simulink model "cv_model_50F"  (R2023a)
settings: Solver=ode23t  StartTime=0  StopTime=5040  FixedStep=0.0005  MaxStep=.01  RelTol=1e-4
model workspace (MAT data in the model file):
  test = 0
values from neighbouring files (symbols this model uses):
  A_cheb_09_1 = [-9.45889157397 1 0 0 0 0 0 0 0 -116.684730988 0 1 ... (81 elements, 9x9)]    [input_reflex_filters.mat]
  B_cheb_09_1 = [1 0 0 0 0 0 0 0 0]    [input_reflex_filters.mat]
  C_cheb_09_1 = [0 0 0 0 0 0 0 0 151338.279895]    [input_reflex_filters.mat]
libraries: SignalEditorBlockLib x4, simulink_extras x2
(part 1 of 3)
settings Model: ExtModeTrigMode=oneshot  Creator=samar  LastModifiedBy=Rich
settings SolverCC: AlgebraicLoopSolver=TrustRegion
settings DataIOCC: SaveFormat=Array  SignalLoggingSaveFormat=ModelDataLogs  ReturnWorkspaceOutputs=off  SignalLoggingName=sigsOut
settings OptimizationCC: BooleanDataType=off  InitFltsAndDblsToZero=on  LifeSpan=inf
settings DebuggingCC: ConsistencyChecking=warning  SaveWithParameterizedLinksMsg=none  UnderspecifiedInitializationDetection=Classic  MergeDetectMultiDrivingBlocksExec=none  SignalResolutionControl=TryResolveAllWithWarning  MultiTaskDSMMsg=warning  MultiTaskCondExecSysMsg=none  FcnCallInpInsideContextMsg=warning  SFUnexpectedBacktrackingDiag=warning  SFNoUnconditionalDefaultTransitionDiag=warning  SFExecutionAtInitializationDiag=none  ArithmeticOperatorsInVariantConditions=warning
settings HardwareCC: ProdBitPerPointer=32  ProdBitPerSizeT=32  ProdBitPerPtrDiffT=32  ProdLargestAtomicFloat=None  ProdIntDivRoundTo=Undefined  ProdEndianess=Unspecified  ProdWordSize=32  ProdHWDeviceType=32-bit Generic  TargetUnknown=on
settings ModelReferenceCC: EnableRefExpFcnMdlSchedulingChecks=on  PropagateSignalLabelsOutOfModel=off
settings SFSimCC: SimUseLocalCustomCode=off  CustomCodeUndefinedFunction=UseInterfaceOnly
settings RTWCC: TemplateMakefile=grt_unix.tmf  RTWUseLocalCustomCode=off  DLArmComputeVersion=19.05
settings CodeAppCC: StateflowObjectComments=on
settings GRTTargetCC: TargetFcnLib=ansi_tfl_tmw.mat  TargetLangStandard=C89/C90 (ANSI)  ModelReferenceCompliant=off  CombineOutputUpdateFcns=off  MatFileLogging=off  GRTInterface=on
settings ConfigComp: CovMetricSettings=dw  CovSaveCumulativeToWorkspaceVar=on  CovSaveSingleToWorkspaceVar=on  CovExternalEMLEnable=off  CovSFcnEnable=off

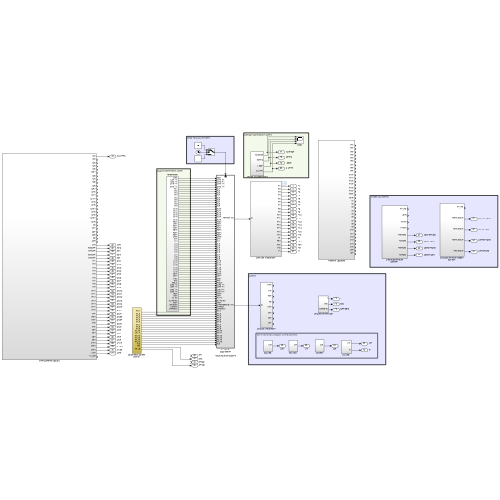
[thumbnail: Simulink's stored preview of the top-level diagram]
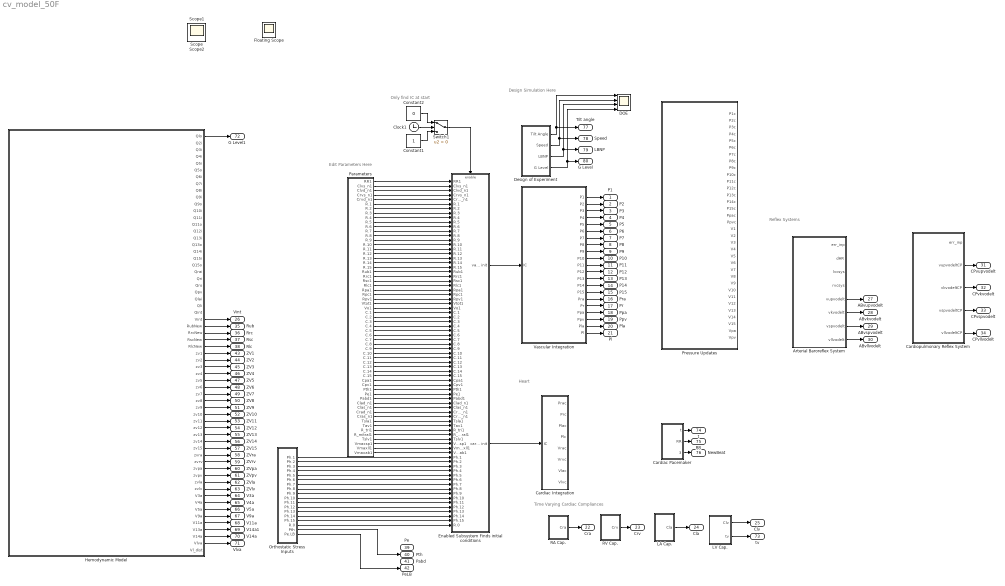
== system cv_model_50F ==
  note: Design Simulation Here
  note: Edit Parameters Here
  note: Reflex Systems
  note: Heart
  note: Time Varying Cardiac Compliances
  note: Only find IC at start
  Arterial Baroreflex System : Subsystem
  Cardiac Integration : Subsystem
  Cardiac Pacemaker : Subsystem
  Cardiopulmonary Reflex System : Subsystem
  Clock1 : Clock
  Constant1 : Constant
  Constant2 : Constant  Value=0
  DOE : Scope  NumInputPorts=4
  Design of Experiment : Subsystem
  Enabled Subsystem Finds initial conditions : Subsystem  TreatAsAtomicUnit=on
  Hemodynamic Model : Subsystem
  LA Cap. : Subsystem
  LV Cap. : Subsystem
  Orthostatic Stress Inputs : Subsystem
  Parameters : Subsystem
  Pressure Updates : Subsystem
  RA Cap. : Subsystem
  RV Cap. : Subsystem
  Switch1 : Switch  Criteria=u2 > Threshold
  Vascular Integration : Subsystem
  P1 : Outport
  P2 : Outport  Port=2
  P3 : Outport  Port=3
  P4 : Outport  Port=4
  P5 : Outport  Port=5
  P6 : Outport  Port=6
  P7 : Outport  Port=7
  P8 : Outport  Port=8
  P9 : Outport  Port=9
  P10 : Outport  Port=10
  P11 : Outport  Port=11
  P12 : Outport  Port=12
  P13 : Outport  Port=13
  P14 : Outport  Port=14
  P15 : Outport  Port=15
  Pra : Outport  Port=16
  Pr : Outport  Port=17
  Ppa : Outport  Port=18
  Ppv : Outport  Port=19
  Pla : Outport  Port=20
  Pl : Outport  Port=21
  Cra : Outport  Port=22
  Crv : Outport  Port=23
  Cla : Outport  Port=24
  Clv : Outport  Port=25
  Vint : Outport  Port=26
  ABvupvodelt : Outport  Port=27
  ABvkvodelt : Outport  Port=28
  ABvspvodelt : Outport  Port=29
  ABvllvodelt : Outport  Port=30
  CPvupvodelt : Outport  Port=31
  CPvkvodelt : Outport  Port=32
  CPvspvodelt : Outport  Port=33
  CPvllvodelt : Outport  Port=34
  Rub : Outport  Port=35
  Rrc : Outport  Port=36
  Rsc : Outport  Port=37
  Rlc : Outport  Port=38
  Pe : Outport  Port=39
  Pth : Outport  Port=40
  Pabd : Outport  Port=41
  PeLB : Outport  Port=42
  ZV1 : Outport  Port=43
  ZV2 : Outport  Port=44
  ZV3 : Outport  Port=45
  ZV4 : Outport  Port=46
  ZV5 : Outport  Port=47
  ZV6 : Outport  Port=48
  ZV7 : Outport  Port=49
  ZV8 : Outport  Port=50
  ZV9 : Outport  Port=51
  ZV10 : Outport  Port=52
  ZV11 : Outport  Port=53
  ZV12 : Outport  Port=54
  ZV13 : Outport  Port=55
  ZV14 : Outport  Port=56
  ZV15 : Outport  Port=57
  ZVra : Outport  Port=58
  ZVrv : Outport  Port=59
  ZVpa : Outport  Port=60
  ZVpv : Outport  Port=61
  ZVla : Outport  Port=62
  ZVlv : Outport  Port=63
  V3a : Outport  Port=64
  V4a : Outport  Port=65
  V5a : Outport  Port=66
  V9a : Outport  Port=67
  V11a : Outport  Port=68
  V14a1 : Outport  Port=69
  V14a : Outport  Port=70
  Vlva : Outport  Port=71
  G Level1 : Outport  Port=72
  tv : Outport  Port=73
  t : Outport  Port=74
  RR : Outport  Port=75
  NewBeat : Outport  Port=76
  Tilt angle : Outport  Port=77
  Speed : Outport  Port=78
  LBNP : Outport  Port=79
  G Level : Outport  Port=80
  Floating Scope : Scope
  Scope : Scope
  Scope1 : Scope
  Scope2 : Scope
  wires:
  Enabled Subsystem Finds initial conditions/2(cardiac init) -> Cardiac Integration/1(IC)
  Enabled Subsystem Finds initial conditions/1(vascular init) -> Vascular Integration/1(IC)
  Constant2/1 -> Switch1/1
  Clock1/1 -> Switch1/2
  Constant1/1 -> Switch1/3
  Vascular Integration/21(Pl) -> Pl/1
  Vascular Integration/17(Pr) -> Pr/1
  Vascular Integration/18(Ppa) -> Ppa/1
  Vascular Integration/19(Ppv) -> Ppv/1
  Vascular Integration/1(P1) -> P1/1
  Vascular Integration/2(P2) -> P2/1
  Vascular Integration/3(P3) -> P3/1
  Vascular Integration/4(P4) -> P4/1
  Vascular Integration/5(P5) -> P5/1
  Vascular Integration/6(P6) -> P6/1
  Vascular Integration/7(P7) -> P7/1
  Vascular Integration/8(P8) -> P8/1
  Vascular Integration/9(P9) -> P9/1
  Vascular Integration/10(P10) -> P10/1
  Vascular Integration/11(P11) -> P11/1
  Vascular Integration/12(P12) -> P12/1
  Vascular Integration/13(P13) -> P13/1
  Vascular Integration/14(P14) -> P14/1
  Vascular Integration/15(P15) -> P15/1
  Switch1/1 -> Enabled Subsystem Finds initial conditions/Enable
  Arterial Baroreflex System/7(vspvodelt) -> ABvspvodelt/1
  Arterial Baroreflex System/5(vupvodelt) -> ABvupvodelt/1
  Cardiopulmonary Reflex System/4(vspvodeltCP) -> CPvspvodelt/1
  Cardiopulmonary Reflex System/3(vkvodeltCP) -> CPvkvodelt/1
  Cardiopulmonary Reflex System/5(vllvodeltCP) -> CPvllvodelt/1
  RA Cap./1(Cra) -> Cra/1
  LA Cap./1(Cla) -> Cla/1
  Cardiac Pacemaker/1(t) -> t/1
  LV Cap./1(Clv) -> Clv/1
  LV Cap./2(tv) -> tv/1
  RV Cap./1(Crv) -> Crv/1
  Vascular Integration/16(Pra) -> Pra/1
  Vascular Integration/20(Pla) -> Pla/1
  Arterial Baroreflex System/6(vkvodelt) -> ABvkvodelt/1
  Arterial Baroreflex System/8(vllvodelt) -> ABvllvodelt/1
  Cardiopulmonary Reflex System/2(vupvodeltCP) -> CPvupvodelt/1
  Orthostatic Stress Inputs/17(Pth) -> Pth/1
  Cardiac Pacemaker/2(RR) -> RR/1
  Cardiac Pacemaker/3(NewBeat) -> NewBeat/1
  Orthostatic Stress Inputs/18(Pe.LB) -> PeLB/1
  Hemodynamic Model/58(V11a) -> V11a/1
  Hemodynamic Model/32(RlcNew) -> Rlc/1
  Hemodynamic Model/57(V9a) -> V9a/1
  Hemodynamic Model/30(RrcNew) -> Rrc/1
  Hemodynamic Model/54(V3a) -> V3a/1
  Hemodynamic Model/31(RscNew) -> Rsc/1
  Hemodynamic Model/60(V14a) -> V14a/1
  Hemodynamic Model/61(Vlva) -> Vlva/1
  Hemodynamic Model/55(V4a) -> V4a/1
  Hemodynamic Model/29(RubNew) -> Rub/1
  Hemodynamic Model/56(V5a) -> V5a/1
  Design of Experiment/3(LBNP) -> DOE/3, LBNP/1
  Design of Experiment/1(Tilt Angle) -> Tilt angle/1, DOE/1
  Hemodynamic Model/28(Vint) -> Vint/1
  Design of Experiment/4(G Level) -> DOE/4, G Level/1
  Design of Experiment/2(Speed) -> DOE/2, Speed/1
  Parameters/49(Pabd1) -> Enabled Subsystem Finds initial conditions/49(Pabd1)
  Parameters/50(Clad_n1) -> Enabled Subsystem Finds initial conditions/50(Clad_n1)
  Parameters/51(Clas_n1) -> Enabled Subsystem Finds initial conditions/51(Clas_n1)
  Parameters/52(Crad_n1) -> Enabled Subsystem Finds initial conditions/52(Crad_n1)
  Parameters/53(Cras_n1) -> Enabled Subsystem Finds initial conditions/53(Cras_n1)
  Parameters/54(Tsla1) -> Enabled Subsystem Finds initial conditions/54(Tsla1)
  Parameters/55(Tav1) -> Enabled Subsystem Finds initial conditions/55(Tav1)
  Parameters/56(R_tri1) -> Enabled Subsystem Finds initial conditions/56(R_tri1)
  Parameters/57(R_mitral1) -> Enabled Subsystem Finds initial conditions/57(R_mitral1)
  Parameters/58(Tslv1) -> Enabled Subsystem Finds initial conditions/58(Tslv1)
  Parameters/59(Vmaxsp1) -> Enabled Subsystem Finds initial conditions/59(Vmaxsp1)
  Parameters/60(Vmaxll1) -> Enabled Subsystem Finds initial conditions/60(Vmaxll1)
  Parameters/61(Vmaxab1) -> Enabled Subsystem Finds initial conditions/61(Vmaxab1)
  Orthostatic Stress Inputs/1(Ph.1) -> Enabled Subsystem Finds initial conditions/62(Ph.1)
  Orthostatic Stress Inputs/2(Ph.2) -> Enabled Subsystem Finds initial conditions/63(Ph.2)
  Orthostatic Stress Inputs/3(Ph.3) -> Enabled Subsystem Finds initial conditions/64(Ph.3)
  Orthostatic Stress Inputs/4(Ph.4) -> Enabled Subsystem Finds initial conditions/65(Ph.4)
  Orthostatic Stress Inputs/5(Ph.5) -> Enabled Subsystem Finds initial conditions/66(Ph.5)
  Orthostatic Stress Inputs/6(Ph.6) -> Enabled Subsystem Finds initial conditions/67(Ph.6)
  Orthostatic Stress Inputs/7(Ph.7) -> Enabled Subsystem Finds initial conditions/68(Ph.7)
  Orthostatic Stress Inputs/8(Ph.8) -> Enabled Subsystem Finds initial conditions/69(Ph.8)
  Orthostatic Stress Inputs/9(Ph.9) -> Enabled Subsystem Finds initial conditions/70(Ph.9)
  Orthostatic Stress Inputs/10(Ph.10) -> Enabled Subsystem Finds initial conditions/71(Ph.10)
  Orthostatic Stress Inputs/11(Ph.11) -> Enabled Subsystem Finds initial conditions/72(Ph.11)
  Orthostatic Stress Inputs/12(Ph.12) -> Enabled Subsystem Finds initial conditions/73(Ph.12)
  Orthostatic Stress Inputs/13(Ph.13) -> Enabled Subsystem Finds initial conditions/74(Ph.13)
  Orthostatic Stress Inputs/14(Ph.14) -> Enabled Subsystem Finds initial conditions/75(Ph.14)
  Orthostatic Stress Inputs/15(Ph.15) -> Enabled Subsystem Finds initial conditions/76(Ph.15)
  Orthostatic Stress Inputs/16(R.0) -> Enabled Subsystem Finds initial conditions/77(R.0)
  Parameters/1(RR1) -> Enabled Subsystem Finds initial conditions/1(RR1)
  Parameters/2(Clvs_n1) -> Enabled Subsystem Finds initial conditions/2(Clvs_n1)
  Parameters/3(Clvd_n1) -> Enabled Subsystem Finds initial conditions/3(Clvd_n1)
  Parameters/4(Crvs_n1) -> Enabled Subsystem Finds initial conditions/4(Crvs_n1)
  Parameters/5(Crvd_n1) -> Enabled Subsystem Finds initial conditions/5(Crvd_n1)
  Parameters/6(R.1) -> Enabled Subsystem Finds initial conditions/6(R.1)
  Parameters/7(R.2) -> Enabled Subsystem Finds initial conditions/7(R.2)
  Parameters/8(R.3) -> Enabled Subsystem Finds initial conditions/8(R.3)
  Parameters/9(R.4) -> Enabled Subsystem Finds initial conditions/9(R.4)
  Parameters/10(R.5) -> Enabled Subsystem Finds initial conditions/10(R.5)
  Parameters/11(R.6) -> Enabled Subsystem Finds initial conditions/11(R.6)
  Parameters/12(R.7) -> Enabled Subsystem Finds initial conditions/12(R.7)
  Parameters/13(R.8) -> Enabled Subsystem Finds initial conditions/13(R.8)
  Parameters/14(R.9) -> Enabled Subsystem Finds initial conditions/14(R.9)
  Parameters/15(R.10) -> Enabled Subsystem Finds initial conditions/15(R.10)
  Parameters/16(R.11) -> Enabled Subsystem Finds initial conditions/16(R.11)
  Parameters/17(R.12) -> Enabled Subsystem Finds initial conditions/17(R.12)
  Parameters/18(R.13) -> Enabled Subsystem Finds initial conditions/18(R.13)
  Parameters/19(R.14) -> Enabled Subsystem Finds initial conditions/19(R.14)
  Parameters/20(R.15) -> Enabled Subsystem Finds initial conditions/20(R.15)
  Parameters/21(Rub1) -> Enabled Subsystem Finds initial conditions/21(Rub1)
  Parameters/22(Rrc1) -> Enabled Subsystem Finds initial conditions/22(Rrc1)
  Parameters/23(Rsc1) -> Enabled Subsystem Finds initial conditions/23(Rsc1)
  Parameters/24(Rlc1) -> Enabled Subsystem Finds initial conditions/24(Rlc1)
  Parameters/25(Rpa1) -> Enabled Subsystem Finds initial conditions/25(Rpa1)
  Parameters/26(Rpc1) -> Enabled Subsystem Finds initial conditions/26(Rpc1)
  Parameters/27(Rpv1) -> Enabled Subsystem Finds initial conditions/27(Rpv1)
  Parameters/28(Vtot1) -> Enabled Subsystem Finds initial conditions/28(Vtot1)
  Parameters/29(Vo1) -> Enabled Subsystem Finds initial conditions/29(Vo1)
  Parameters/30(C.1) -> Enabled Subsystem Finds initial conditions/30(C.1)
  Parameters/31(C.2) -> Enabled Subsystem Finds initial conditions/31(C.2)
  Parameters/32(C.3) -> Enabled Subsystem Finds initial conditions/32(C.3)
  Parameters/33(C.4) -> Enabled Subsystem Finds initial conditions/33(C.4)
  Parameters/34(C.5) -> Enabled Subsystem Finds initial conditions/34(C.5)
  Parameters/35(C.6) -> Enabled Subsystem Finds initial conditions/35(C.6)
  Parameters/36(C.7) -> Enabled Subsystem Finds initial conditions/36(C.7)
  Parameters/37(C.8) -> Enabled Subsystem Finds initial conditions/37(C.8)
  Parameters/38(C.9) -> Enabled Subsystem Finds initial conditions/38(C.9)
  Parameters/39(C.10) -> Enabled Subsystem Finds initial conditions/39(C.10)
  Parameters/40(C.11) -> Enabled Subsystem Finds initial conditions/40(C.11)
  Parameters/41(C.12) -> Enabled Subsystem Finds initial conditions/41(C.12)
  Parameters/42(C.13) -> Enabled Subsystem Finds initial conditions/42(C.13)
  Parameters/43(C.14) -> Enabled Subsystem Finds initial conditions/43(C.14)
  Parameters/44(C.15) -> Enabled Subsystem Finds initial conditions/44(C.15)
  Parameters/45(Cpa1) -> Enabled Subsystem Finds initial conditions/45(Cpa1)
  Parameters/46(Cpv1) -> Enabled Subsystem Finds initial conditions/46(Cpv1)
  Parameters/47(Pth1) -> Enabled Subsystem Finds initial conditions/47(Pth1)
  Parameters/48(Pe1) -> Enabled Subsystem Finds initial conditions/48(Pe1)
  Hemodynamic Model/33(zv1) -> ZV1/1
  Hemodynamic Model/34(zv2) -> ZV2/1
  Hemodynamic Model/35(zv3) -> ZV3/1
  Hemodynamic Model/36(zv4) -> ZV4/1
  Hemodynamic Model/37(zv5) -> ZV5/1
  Hemodynamic Model/38(zv6) -> ZV6/1
  Hemodynamic Model/39(zv7) -> ZV7/1
  Hemodynamic Model/40(zv8) -> ZV8/1
  Hemodynamic Model/41(zv9) -> ZV9/1
  Hemodynamic Model/42(zv10) -> ZV10/1
  Hemodynamic Model/43(zv11) -> ZV11/1
  Hemodynamic Model/44(zv12) -> ZV12/1
  Hemodynamic Model/45(zv13) -> ZV13/1
  Hemodynamic Model/46(zv14) -> ZV14/1
  Hemodynamic Model/47(zv15) -> ZV15/1
  Hemodynamic Model/48(zvra) -> ZVra/1
  Hemodynamic Model/49(zvrv) -> ZVrv/1
  Hemodynamic Model/50(zvpa) -> ZVpa/1
  Hemodynamic Model/51(zvpv) -> ZVpv/1
  Hemodynamic Model/52(zvla) -> ZVla/1
  Hemodynamic Model/53(zvlv) -> ZVlv/1
  Hemodynamic Model/59(V13a) -> V14a1/1
  Hemodynamic Model/1(Qlo) -> G Level1/1

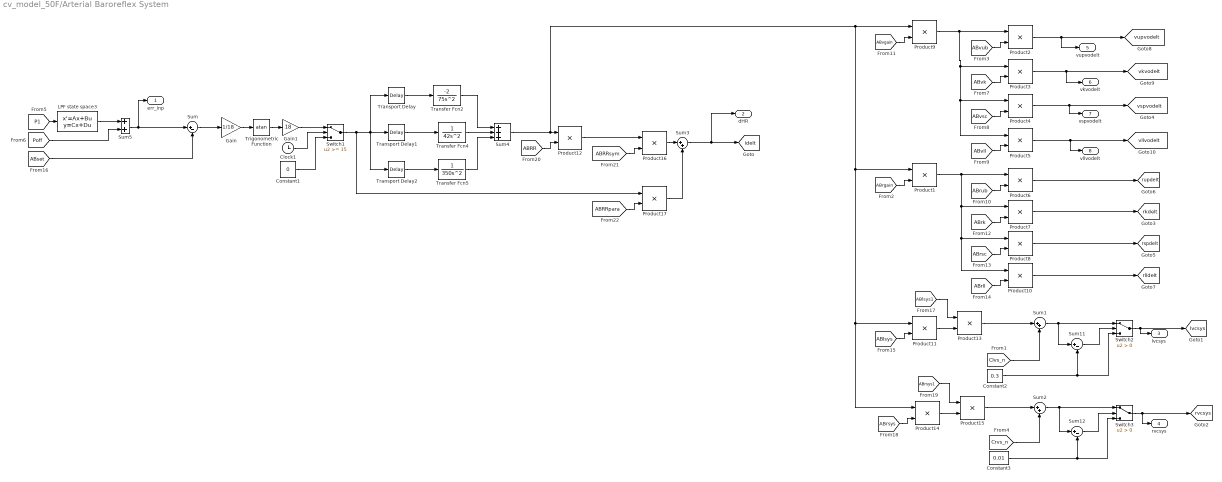
== system cv_model_50F/Arterial Baroreflex System ==
  Clock1 : Clock
  Constant1 : Constant  Value=0
  Constant2 : Constant  Value=0.3
  Constant3 : Constant  Value=0.01
  Gain : Gain  Gain=1/18  SaturateOnIntegerOverflow=on  OutDataTypeStr=Inherit: Same as input  ParamDataTypeStr=Inherit: Same as input
  Gain1 : Gain  Gain=18  SaturateOnIntegerOverflow=on  OutDataTypeStr=Inherit: Same as input  ParamDataTypeStr=Inherit: Same as input
  LPF state space3 : StateSpace  A=A_cheb_09_1  B=B_cheb_09_1  C=C_cheb_09_1  D=0  InitialCondition=[0 0 0 0 0 0 0 0 91/C_cheb_09_1(9)]
  Product{1..17} (17 alike) : Product  Inputs=**  SaturateOnIntegerOverflow=on  OutDataTypeStr=Inherit: Same as first input
  Sum : Sum  Inputs=|+-  InputSameDT=on  SaturateOnIntegerOverflow=on  OutDataTypeStr=Inherit: Same as first input
  Sum1 : Sum  Inputs=|++  InputSameDT=on  SaturateOnIntegerOverflow=on  OutDataTypeStr=Inherit: Same as first input
  Sum11 : Sum  Inputs=|+-  InputSameDT=on  SaturateOnIntegerOverflow=on  OutDataTypeStr=Inherit: Same as first input
  Sum12 : Sum  Inputs=|+-  InputSameDT=on  SaturateOnIntegerOverflow=on  OutDataTypeStr=Inherit: Same as first input
  Sum2 : Sum  Inputs=|++  InputSameDT=on  SaturateOnIntegerOverflow=on  OutDataTypeStr=Inherit: Same as first input
  Sum3 : Sum  Inputs=|++  InputSameDT=on  SaturateOnIntegerOverflow=on  OutDataTypeStr=Inherit: Same as first input
  Sum4 : Sum  Inputs=+++  InputSameDT=on  SaturateOnIntegerOverflow=on  OutDataTypeStr=Inherit: Same as first input
  Sum5 : Sum  InputSameDT=on  SaturateOnIntegerOverflow=on  OutDataTypeStr=Inherit: Same as first input
  Switch1 : Switch  Threshold=15
  Switch2 : Switch  Criteria=u2 > Threshold
  Switch3 : Switch  Criteria=u2 > Threshold
  Transfer Fcn2 : TransferFcn  Numerator=-2  Denominator=[75 0 0]
  Transfer Fcn4 : TransferFcn  Numerator=1  Denominator=[42 0 0 ]
  Transfer Fcn5 : TransferFcn  Numerator=1  Denominator=[350 0 0 ]
  Transport Delay : TransportDelay  DelayTime=5
  Transport Delay1 : TransportDelay  DelayTime=2
  Transport Delay2 : TransportDelay  DelayTime=30  BufferSize=6144
  Trigonometric Function : Trigonometry  Operator=atan
  err_inp : Outport
  dHR : Outport  Port=2
  lvcsys : Outport  Port=3
  rvcsys : Outport  Port=4
  vupvodelt : Outport  Port=5
  vkvodelt : Outport  Port=6
  vspvodelt : Outport  Port=7
  vllvodelt : Outport  Port=8
  tag scope: idelt=global, lvcsys=global, rkdelt=global, rlldelt=global, rspdelt=global, rupdelt=global, rvcsys=global, vkvodelt=global, vllvodelt=global, vspvodelt=global, vupvodelt=global
  wires:
  Sum/1 -> Gain/1
  Product15/1 -> Sum2/1
  Product13/1 -> Sum1/1
  Sum1/1 -> Sum11/1, Switch2/1
  Product7/1 -> [rkdelt]
  Product4/1 -> [vspvodelt], vspvodelt/1
  [Crvs_n] -> Sum2/2
  [Clvs_n] -> Sum1/2
  Trigonometric Function/1 -> Gain1/1
  Product10/1 -> [rlldelt]
  Product6/1 -> [rupdelt]
  Product8/1 -> [rspdelt]
  Product2/1 -> vupvodelt/1, [vupvodelt]
  Product3/1 -> vkvodelt/1, [vkvodelt]
  Product5/1 -> vllvodelt/1, [vllvodelt]
  Product9/1 -> Product2/1, Product3/1, Product4/1, Product5/1
  Product1/1 -> Product6/1, Product7/1, Product8/1, Product10/1
  Sum4/1 -> Product12/1, Product9/1, Product1/1, Product14/1, Product11/1
  Gain1/1 -> Switch1/1
  Product16/1 -> Sum3/1
  Sum3/1 -> [idelt], dHR/1
  Product17/1 -> Sum3/2
  Clock1/1 -> Switch1/2
  Constant1/1 -> Switch1/3
  Switch1/1 -> Product17/1, Transport Delay1/1, Transport Delay/1, Transport Delay2/1
  Gain/1 -> Trigonometric Function/1
  Sum5/1 -> err_inp/1, Sum/1
  Sum11/1 -> Switch2/2
  Constant2/1 -> Switch2/3, Sum11/2
  Switch2/1 -> [lvcsys], lvcsys/1
  Sum2/1 -> Switch3/1, Sum12/1
  Sum12/1 -> Switch3/2
  Constant3/1 -> Switch3/3, Sum12/2
  Switch3/1 -> [rvcsys], rvcsys/1
  [P1] -> LPF state space3/1
  Transport Delay/1 -> Transfer Fcn2/1
  Transport Delay1/1 -> Transfer Fcn4/1
  Transport Delay2/1 -> Transfer Fcn5/1
  Transfer Fcn2/1 -> Sum4/1
  Transfer Fcn4/1 -> Sum4/2
  Transfer Fcn5/1 -> Sum4/3
  LPF state space3/1 -> Sum5/1
  [Poff] -> Sum5/2
  [ABset] -> Sum/2
  [ABvgain] -> Product9/2
  [ABrgain] -> Product1/2
  [ABvub] -> Product2/2
  [ABvk] -> Product3/2
  [ABvsc] -> Product4/2
  [ABvll] -> Product5/2
  [ABrub] -> Product6/2
  [ABrk] -> Product7/2
  [ABrsc] -> Product8/2
  [ABrll] -> Product10/2
  [ABlsys] -> Product11/2
  Product11/1 -> Product13/2
  [ABlsys1] -> Product13/1
  [ABrsys1] -> Product15/1
  [ABrsys] -> Product14/2
  Product14/1 -> Product15/2
  [ABRR] -> Product12/2
  [ABRRsym] -> Product16/2
  Product12/1 -> Product16/1
  [ABRRpara] -> Product17/2

== system cv_model_50F/Cardiac Integration ==
  IC : Inport
  Demux1 : Demux
      settings: DisplayOption=none
  Integrator1 : Integrator  InitialConditionSource=external  InitialCondition=[220.105 68.078]
  Math Function1 : Math  Operator=reciprocal  SignedPower=on
  Math Function3 : Math  Operator=reciprocal  SignedPower=on
  Math Function4 : Math  Operator=reciprocal  SignedPower=on
  Mux2 : Mux
  Product : Product  Inputs=*/  SaturateOnIntegerOverflow=on  OutDataTypeStr=Inherit: Same as first input
  Product1 : Product  SaturateOnIntegerOverflow=on  OutDataTypeStr=Inherit: Same as first input
  Product2 : Product  SaturateOnIntegerOverflow=on  OutDataTypeStr=Inherit: Same as first input
  Product3 : Product  SaturateOnIntegerOverflow=on  OutDataTypeStr=Inherit: Same as first input
  Product4 : Product  Inputs=*/  SaturateOnIntegerOverflow=on  OutDataTypeStr=Inherit: Same as first input
  Sum{1..4} (4 alike) : Sum  InputSameDT=on  SaturateOnIntegerOverflow=on  OutDataTypeStr=Inherit: Same as first input
  Switch2 : Switch  Criteria=u2 > Threshold
  Prac : Outport
  Prc : Outport  Port=2
  Plac : Outport  Port=3
  Plc : Outport  Port=4
  Vrac : Outport  Port=5
  Vrvc : Outport  Port=6
  Vlac : Outport  Port=7
  Vlvc : Outport  Port=8
  tag scope: Pl=global, Pla=global, Pr=global, Pra=global, Vl_dist=global, Vla=global, Vra=global, Vrv=global
  wires:
  Mux2/1 -> Integrator1/1
  [dVl] -> Mux2/1
  [dVr] -> Mux2/2
  Integrator1/1 -> Demux1/1
  [Crv] -> Math Function1/1
  Math Function1/1 -> Product1/2
  Demux1/2 -> Product1/1, [Vrv], Vrvc/1
  Product1/1 -> Sum1/1, Prc/1
  [Pth] -> Sum1/2
  Sum1/1 -> [Pr]
  [Pth] -> Sum2/2
  Sum2/1 -> [Pl]
  IC/1 -> Integrator1/2
  [dVla] -> Mux2/3
  [dVra] -> Mux2/4
  [Cla] -> Math Function3/1
  Math Function3/1 -> Product2/2
  Product2/1 -> Plac/1, Sum3/1
  [Pth] -> Sum3/2
  [Cra] -> Math Function4/1
  Math Function4/1 -> Product3/2
  Product3/1 -> Sum4/1, Prac/1
  [Pth] -> Sum4/2
  Sum4/1 -> [Pra]
  Demux1/4 -> [Vra], Vrac/1, Product3/1
  [Clv] -> Switch2/1
  [ZVlv] -> Product4/1
  [Pcol] -> Product4/2
  Switch2/1 -> Product/2
  Product4/1 -> Switch2/3
  Product/1 -> Plc/1, Sum2/1
  Sum3/1 -> [Pla]
  Demux1/1 -> Switch2/2, Product/1, [Vl_dist], Vlvc/1
  Demux1/3 -> [Vla], Vlac/1, Product2/1

== system cv_model_50F/Cardiac Pacemaker ==
  note: New Beat Logic
  note: Define New RR Interval
  note: Define m(n) = 1/I(n) = 1/(I0 + dI)
  Clock1 : Clock
  Clock2 : Clock
  Constant : Constant  Value=60
  Constant1 : Constant
  Constant2 : Constant  Value=0
  Constant4 : Constant  Value=0
  Divide : Product  Inputs=*/
  Gain1 : Gain  Gain=0.001
  Gain2 : Gain  Gain=0.2
  Gain3 : Gain  Gain=1.5
  Gain4 : Gain  Gain=0.001
  HRVisual : Scope
  Integrator : Integrator  ExternalReset=level  InitialConditionSource=external
  Logical Operator1 : Logic  Inputs=3  OutDataTypeStr=boolean
  Math Function2 : Math  Operator=reciprocal  SignedPower=on
  Memory1 : Memory  InitialCondition=-0.12*sqrt(6/7)-6/7  InheritSampleTime=on
  Memory2 : Memory  InheritSampleTime=on
  Memory3 : Memory  InitialCondition=-0.12*sqrt(6/7)  InheritSampleTime=on
  Memory4 : Memory  InheritSampleTime=on
  Relational Operator : RelationalOperator  OutDataTypeStr=boolean  InputSameDT=off
  Relational Operator1 : RelationalOperator  OutDataTypeStr=boolean  InputSameDT=off
  Relational Operator2 : RelationalOperator  OutDataTypeStr=boolean  InputSameDT=off
  Relational Operator3 : RelationalOperator  Operator=<  OutDataTypeStr=float('double')  InputSameDT=off
  Scope1 : Scope
  Sum1 : Sum  Inputs=+-  InputSameDT=on  SaturateOnIntegerOverflow=on  OutDataTypeStr=Inherit: Same as first input
  Sum11 : Sum  Inputs=+-  InputSameDT=on  SaturateOnIntegerOverflow=on  OutDataTypeStr=Inherit: Same as first input
  Sum2 : Sum  InputSameDT=on  SaturateOnIntegerOverflow=on  OutDataTypeStr=Inherit: Same as first input
  Sum3 : Sum  Inputs=+-  InputSameDT=on  SaturateOnIntegerOverflow=on  OutDataTypeStr=Inherit: Same as first input
  Switch1 : Switch  Threshold=0.5
  Switch2 : Switch  Criteria=u2 > Threshold
  Switch4 : Switch  Criteria=u2 > Threshold  Threshold=0.5
  mult1 : Product  Inputs=*/
  t : Outport
  RR : Outport  Port=2
  NewBeat : Outport  Port=3
  tag scope: NewBeat=global, RR=global, m=global, t=global
  wires:
  Switch4/1 -> Memory3/1, Sum1/1, Sum3/2
  Memory3/1 -> Switch4/3, Switch1/1
  Clock1/1 -> Switch4/1, Sum3/1
  [m] -> Integrator/1
  Integrator/1 -> Relational Operator/1, Sum11/1, Memory4/1
  Relational Operator/1 -> Logical Operator1/1
  Constant1/1 -> Relational Operator/2
  [RR0] -> Sum2/1
  [idelt] -> Sum2/2
  Sum2/1 -> Gain1/1
  Gain1/1 -> Math Function2/1
  Math Function2/1 -> [m]
  Logical Operator1/1 -> Integrator/2
  Relational Operator1/1 -> Logical Operator1/2
  Switch1/1 -> Memory1/1, Sum1/2
  Memory1/1 -> Switch1/3
  Sum1/1 -> [RR], Divide/2, RR/1
  Clock2/1 -> Switch2/2
  mult1/1 -> Switch2/3
  [Tav0] -> mult1/1
  Constant2/1 -> Switch2/1
  Switch2/1 -> Integrator/3
  Sum3/1 -> [t], t/1
  [t] -> Relational Operator1/1
  [RR] -> Gain2/1
  Gain2/1 -> Relational Operator1/2
  Relational Operator2/1 -> Logical Operator1/3
  [Tslv] -> Gain3/1
  Gain3/1 -> Relational Operator2/2
  [tv] -> Relational Operator2/1
  Memory4/1 -> Sum11/2
  Sum11/1 -> Relational Operator3/1
  Relational Operator3/1 -> Memory2/1
  Constant4/1 -> Relational Operator3/2
  [NewBeat] -> Switch1/2, Switch4/2
  Memory2/1 -> NewBeat/1, Scope1/1, [NewBeat]
  Constant/1 -> Divide/1
  Divide/1 -> HRVisual/1
  Gain4/1 -> mult1/2
  [RR0] -> Gain4/1

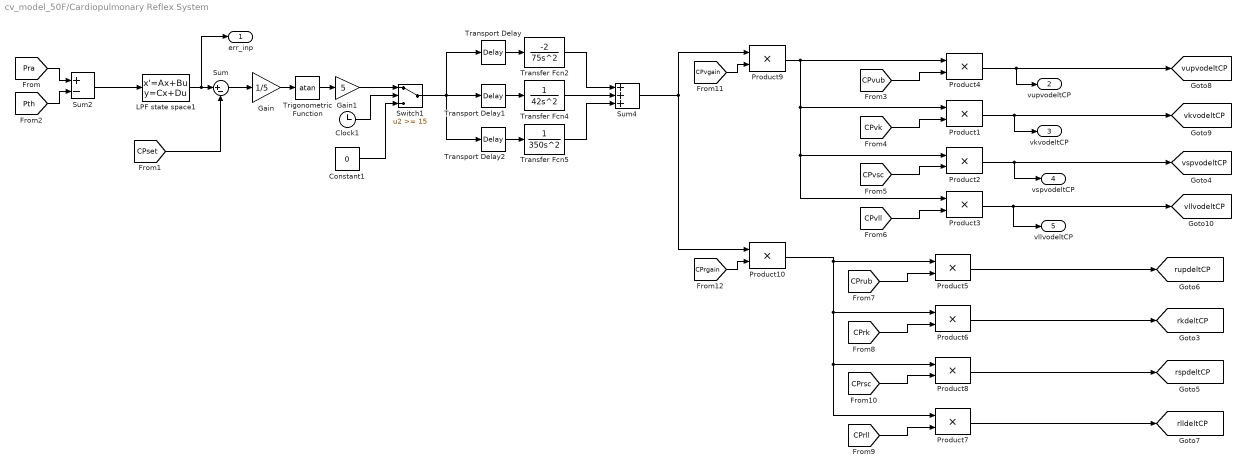
== system cv_model_50F/Cardiopulmonary Reflex System ==
  Clock1 : Clock
  Constant1 : Constant  Value=0
  Gain : Gain  Gain=1/5  SaturateOnIntegerOverflow=on  OutDataTypeStr=Inherit: Same as input  ParamDataTypeStr=Inherit: Same as input
  Gain1 : Gain  Gain=5  SaturateOnIntegerOverflow=on  OutDataTypeStr=Inherit: Same as input  ParamDataTypeStr=Inherit: Same as input
  LPF state space1 : StateSpace  A=A_cheb_09_1  B=B_cheb_09_1  C=C_cheb_09_1  D=0  InitialCondition=[0 0 0 0 0 0 0 0 8.3/C_cheb_09_1(9)]
  Product{1..10} (10 alike) : Product  Inputs=**  SaturateOnIntegerOverflow=on  OutDataTypeStr=Inherit: Same as first input
  Sum : Sum  Inputs=|+-  InputSameDT=on  SaturateOnIntegerOverflow=on  OutDataTypeStr=Inherit: Same as first input
  Sum2 : Sum  Inputs=+-  InputSameDT=on  SaturateOnIntegerOverflow=on  OutDataTypeStr=Inherit: Same as first input
  Sum4 : Sum  Inputs=+++  InputSameDT=on  SaturateOnIntegerOverflow=on  OutDataTypeStr=Inherit: Same as first input
  Switch1 : Switch  Threshold=15
  Transfer Fcn2 : TransferFcn  Numerator=-2  Denominator=[75 0 0]
  Transfer Fcn4 : TransferFcn  Numerator=1  Denominator=[42 0 0 ]
  Transfer Fcn5 : TransferFcn  Numerator=1  Denominator=[350 0 0 ]
  Transport Delay : TransportDelay  DelayTime=5
  Transport Delay1 : TransportDelay  DelayTime=2
  Transport Delay2 : TransportDelay  DelayTime=30  BufferSize=6144
  Trigonometric Function : Trigonometry  Operator=atan
  err_inp : Outport
  vupvodeltCP : Outport  Port=2
  vkvodeltCP : Outport  Port=3
  vspvodeltCP : Outport  Port=4
  vllvodeltCP : Outport  Port=5
  tag scope: rkdeltCP=global, rlldeltCP=global, rspdeltCP=global, rupdeltCP=global, vkvodeltCP=global, vllvodeltCP=global, vspvodeltCP=global, vupvodeltCP=global
  wires:
  Sum/1 -> Gain/1
  [CPset] -> Sum/2
  Gain/1 -> Trigonometric Function/1
  Trigonometric Function/1 -> Gain1/1
  Product6/1 -> [rkdeltCP]
  Product2/1 -> [vspvodeltCP], vspvodeltCP/1
  Product7/1 -> [rlldeltCP]
  Product5/1 -> [rupdeltCP]
  Product8/1 -> [rspdeltCP]
  Product4/1 -> [vupvodeltCP], vupvodeltCP/1
  Product1/1 -> [vkvodeltCP], vkvodeltCP/1
  Product3/1 -> [vllvodeltCP], vllvodeltCP/1
  Product9/1 -> Product4/1, Product1/1, Product3/1, Product2/1
  Product10/1 -> Product5/1, Product6/1, Product7/1, Product8/1
  [Pra] -> Sum2/1
  Gain1/1 -> Switch1/1
  Clock1/1 -> Switch1/2
  Constant1/1 -> Switch1/3
  [Pth] -> Sum2/2
  Sum2/1 -> LPF state space1/1
  LPF state space1/1 -> err_inp/1, Sum/1
  Switch1/1 -> Transport Delay1/1, Transport Delay2/1, Transport Delay/1
  Transfer Fcn5/1 -> Sum4/3
  Transfer Fcn4/1 -> Sum4/2
  Transfer Fcn2/1 -> Sum4/1
  Transport Delay2/1 -> Transfer Fcn5/1
  Transport Delay1/1 -> Transfer Fcn4/1
  Transport Delay/1 -> Transfer Fcn2/1
  Sum4/1 -> Product10/1, Product9/1
  [CPvub] -> Product4/2
  [CPvk] -> Product1/2
  [CPvsc] -> Product2/2
  [CPvll] -> Product3/2
  [CPrub] -> Product5/2
  [CPrk] -> Product6/2
  [CPrll] -> Product7/2
  [CPrsc] -> Product8/2
  [CPvgain] -> Product9/2
  [CPrgain] -> Product10/2

== system cv_model_50F/Design of Experiment ==
  Centrifugation (RPM) : SignalEditorBlockLib/Signal Editor  FileName=doe_src.mat  ActiveScenario=No_Spin  ActiveSignal=RPM  IsBus=off  OutputBusObjectStr=Bus: BusObject  SampleTime=0  ZeroCross=off  OutputAfterFinalValue=Holding final value  Unit=inherit  PreserveSignalName=on  ApplySigPropsToAllScenarios=on
  Gravity Level (g) : SignalEditorBlockLib/Signal Editor  FileName=doe_glevel.mat  ActiveScenario=Earth  ActiveSignal=G Level  IsBus=off  OutputBusObjectStr=Bus: BusObject  SampleTime=0  ZeroCross=off  OutputAfterFinalValue=Holding final value  Unit=inherit  PreserveSignalName=on  ApplySigPropsToAllScenarios=on
  LBNP (mmHg) : SignalEditorBlockLib/Signal Editor  FileName=doe_lbnp.mat  ActiveScenario=Omnibus  ActiveSignal=LBNP Pressure  IsBus=off  OutputBusObjectStr=Bus: BusObject  SampleTime=0  ZeroCross=off  OutputAfterFinalValue=Holding final value  Unit=inherit  PreserveSignalName=on  ApplySigPropsToAllScenarios=on
  Switch Block : Subsystem
  Tilt (degrees) : SignalEditorBlockLib/Signal Editor  FileName=doe_tilt.mat  ActiveScenario=No_Tilt  ActiveSignal=Tilt Angle  IsBus=off  OutputBusObjectStr=Bus: BusObject  SampleTime=0  ZeroCross=off  OutputAfterFinalValue=Holding final value  Unit=inherit  PreserveSignalName=on  ApplySigPropsToAllScenarios=on
  Toggle Switch : ToggleSwitchBlock  LabelPosition=Hide
      settings: Values={{'Centrifugation', 'Tilt'}, [0 1]}
  to rad : Gain  Gain=2*pi/360  SaturateOnIntegerOverflow=on  OutDataTypeStr=Inherit: Same as input  ParamDataTypeStr=Inherit: Same as input
  to rad/s : Gain  Gain=2*pi/60  SaturateOnIntegerOverflow=on  OutDataTypeStr=Inherit: Same as input  ParamDataTypeStr=Inherit: Same as input
  Tilt Angle : Outport
  Speed : Outport  Port=2
  LBNP : Outport  Port=3
  G Level : Outport  Port=4
  tag scope: G_LEVEL=global, P_LNBP=global, P_TA=global, W_RADS=global
  wires:
  Tilt (degrees)/1 -> to rad/1
  LBNP (mmHg)/1 -> LBNP/1, [P_LNBP]
  Gravity Level (g)/1 -> [G_LEVEL], G Level/1
  Centrifugation (RPM)/1 -> to rad/s/1
  to rad/1 -> Switch Block/1(In1)
  to rad/s/1 -> Switch Block/2(In2)
  Switch Block/1(Tilt Angle) -> Tilt Angle/1, [P_TA]
  Switch Block/2(Speed) -> Speed/1, [W_RADS]

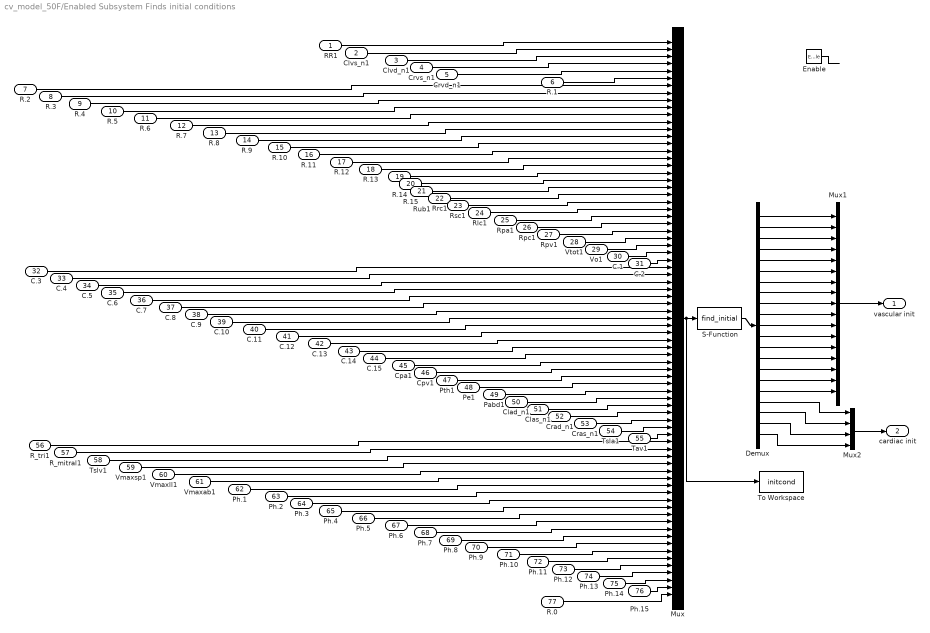
== system cv_model_50F/Enabled Subsystem Finds initial conditions ==
  RR1 : Inport
  Clvs_n1 : Inport  Port=2
  Clvd_n1 : Inport  Port=3
  Crvs_n1 : Inport  Port=4
  Crvd_n1 : Inport  Port=5
  R.1 : Inport  Port=6
  R.2 : Inport  Port=7
  R.3 : Inport  Port=8
  R.4 : Inport  Port=9
  R.5 : Inport  Port=10
  R.6 : Inport  Port=11
  R.7 : Inport  Port=12
  R.8 : Inport  Port=13
  R.9 : Inport  Port=14
  R.10 : Inport  Port=15
  R.11 : Inport  Port=16
  R.12 : Inport  Port=17
  R.13 : Inport  Port=18
  R.14 : Inport  Port=19
  R.15 : Inport  Port=20
  Rub1 : Inport  Port=21
  Rrc1 : Inport  Port=22
  Rsc1 : Inport  Port=23
  Rlc1 : Inport  Port=24
  Rpa1 : Inport  Port=25
  Rpc1 : Inport  Port=26
  Rpv1 : Inport  Port=27
  Vtot1 : Inport  Port=28
  Vo1 : Inport  Port=29
  C.1 : Inport  Port=30
  C.2 : Inport  Port=31
  C.3 : Inport  Port=32
  C.4 : Inport  Port=33
  C.5 : Inport  Port=34
  C.6 : Inport  Port=35
  C.7 : Inport  Port=36
  C.8 : Inport  Port=37
  C.9 : Inport  Port=38
  C.10 : Inport  Port=39
  C.11 : Inport  Port=40
  C.12 : Inport  Port=41
  C.13 : Inport  Port=42
  C.14 : Inport  Port=43
  C.15 : Inport  Port=44
  Cpa1 : Inport  Port=45
  Cpv1 : Inport  Port=46
  Pth1 : Inport  Port=47
  Pe1 : Inport  Port=48
  Pabd1 : Inport  Port=49
  Clad_n1 : Inport  Port=50
  Clas_n1 : Inport  Port=51
  Crad_n1 : Inport  Port=52
  Cras_n1 : Inport  Port=53
  Tsla1 : Inport  Port=54
  Tav1 : Inport  Port=55
  R_tri1 : Inport  Port=56
  R_mitral1 : Inport  Port=57
  Tslv1 : Inport  Port=58
  Vmaxsp1 : Inport  Port=59
  Vmaxll1 : Inport  Port=60
  Vmaxab1 : Inport  Port=61
  Ph.1 : Inport  Port=62
  Ph.2 : Inport  Port=63
  Ph.3 : Inport  Port=64
  Ph.4 : Inport  Port=65
  Ph.5 : Inport  Port=66
  Ph.6 : Inport  Port=67
  Ph.7 : Inport  Port=68
  Ph.8 : Inport  Port=69
  Ph.9 : Inport  Port=70
  Ph.10 : Inport  Port=71
  Ph.11 : Inport  Port=72
  Ph.12 : Inport  Port=73
  Ph.13 : Inport  Port=74
  Ph.14 : Inport  Port=75
  Ph.15 : Inport  Port=76
  R.0 : Inport  Port=77
  Enable : EnablePort  ShowOutputPort=on
  Demux : Demux  Outputs=21
      settings: DisplayOption=none
  Mux : Mux  Inputs=77
  Mux1 : Mux  Inputs=17
  Mux2 : Mux
  S-Function : S-Function  FunctionName=find_initial  SFunctionDeploymentMode=off  EnableBusSupport=off
  To Workspace : ToWorkspace  VariableName=initcond  SampleTime=-1
  vascular init : Outport
  cardiac init : Outport  Port=2
  wires:
  Mux/1 -> S-Function/1, To Workspace/1
  S-Function/1 -> Demux/1
  Mux1/1 -> vascular init/1
  Mux2/1 -> cardiac init/1
  RR1/1 -> Mux/1
  Clvs_n1/1 -> Mux/2
  Clvd_n1/1 -> Mux/3
  Crvs_n1/1 -> Mux/4
  Crvd_n1/1 -> Mux/5
  R.1/1 -> Mux/6
  R.2/1 -> Mux/7
  R.3/1 -> Mux/8
  R.4/1 -> Mux/9
  R.5/1 -> Mux/10
  R.6/1 -> Mux/11
  R.7/1 -> Mux/12
  R.8/1 -> Mux/13
  R.9/1 -> Mux/14
  R.10/1 -> Mux/15
  R.11/1 -> Mux/16
  R.12/1 -> Mux/17
  R.13/1 -> Mux/18
  R.14/1 -> Mux/19
  R.15/1 -> Mux/20
  Rub1/1 -> Mux/21
  Rrc1/1 -> Mux/22
  Rsc1/1 -> Mux/23
  Rlc1/1 -> Mux/24
  Rpa1/1 -> Mux/25
  Rpc1/1 -> Mux/26
  Rpv1/1 -> Mux/27
  Vtot1/1 -> Mux/28
  Vo1/1 -> Mux/29
  C.1/1 -> Mux/30
  C.2/1 -> Mux/31
  C.3/1 -> Mux/32
  C.4/1 -> Mux/33
  C.5/1 -> Mux/34
  C.6/1 -> Mux/35
  C.7/1 -> Mux/36
  C.8/1 -> Mux/37
  C.9/1 -> Mux/38
  C.10/1 -> Mux/39
  C.11/1 -> Mux/40
  C.12/1 -> Mux/41
  C.13/1 -> Mux/42
  C.14/1 -> Mux/43
  C.15/1 -> Mux/44
  Cpa1/1 -> Mux/45
  Cpv1/1 -> Mux/46
  Pth1/1 -> Mux/47
  Pe1/1 -> Mux/48
  Clad_n1/1 -> Mux/50
  Clas_n1/1 -> Mux/51
  Crad_n1/1 -> Mux/52
  Cras_n1/1 -> Mux/53
  Tsla1/1 -> Mux/54
  Tav1/1 -> Mux/55
  R_tri1/1 -> Mux/56
  R_mitral1/1 -> Mux/57
  Tslv1/1 -> Mux/58
  Vmaxsp1/1 -> Mux/59
  Vmaxll1/1 -> Mux/60
  Vmaxab1/1 -> Mux/61
  Pabd1/1 -> Mux/49
  Ph.1/1 -> Mux/62
  Ph.2/1 -> Mux/63
  Demux/18 -> Mux2/1
  Demux/19 -> Mux2/2
  Demux/1 -> Mux1/1
  Demux/2 -> Mux1/2
  Demux/3 -> Mux1/3
  Demux/5 -> Mux1/5
  Demux/6 -> Mux1/6
  Demux/7 -> Mux1/7
  Demux/8 -> Mux1/8
  Demux/9 -> Mux1/9
  Demux/10 -> Mux1/10
  Demux/11 -> Mux1/11
  Demux/12 -> Mux1/12
  Demux/13 -> Mux1/13
  Demux/14 -> Mux1/14
  Demux/15 -> Mux1/15
  Demux/16 -> Mux1/16
  Demux/17 -> Mux1/17
  Enable/1 -> ?
  Ph.3/1 -> Mux/64
  Demux/20 -> Mux2/3
  Demux/21 -> Mux2/4
  Ph.4/1 -> Mux/65
  Ph.5/1 -> Mux/66
  Ph.6/1 -> Mux/67
  Ph.7/1 -> Mux/68
  Ph.8/1 -> Mux/69
  Ph.9/1 -> Mux/70
  Ph.10/1 -> Mux/71
  Ph.11/1 -> Mux/72
  Ph.12/1 -> Mux/73
  Ph.13/1 -> Mux/74
  Ph.14/1 -> Mux/75
  Ph.15/1 -> Mux/76
  Demux/4 -> Mux1/4
  R.0/1 -> Mux/77
